simulink model "fromworkspace_test"  (Simulink 8.4)
settings: Solver=VariableStepDiscrete  StartTime=0.0  StopTime=5  MaxStep=1  RelTol=1e-3
settings Model: Creator=arnaud  LastModifiedBy=arnaud
settings DataIOCC: ExternalInput=xin  SaveFormat=Structure

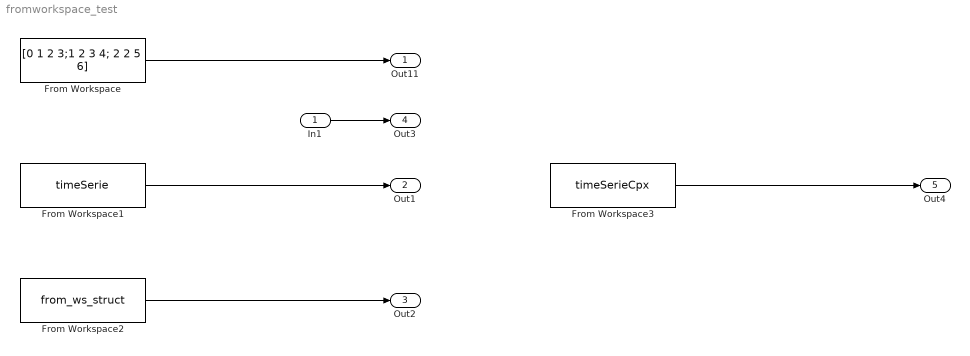
== system fromworkspace_test ==
  In1 : Inport
  From Workspace : FromWorkspace  VariableName=[0 1 2 3;1 2 3 4; 2 2 5 6]  SampleTime=0
  From Workspace1 : FromWorkspace  VariableName=timeSerie  SampleTime=0
  From Workspace2 : FromWorkspace  VariableName=from_ws_struct  OutDataTypeStr=double  SampleTime=0
  From Workspace3 : FromWorkspace  VariableName=timeSerieCpx  SampleTime=0
  Out11 : Outport
  Out1 : Outport  Port=2
  Out2 : Outport  Port=3
  Out3 : Outport  Port=4
  Out4 : Outport  Port=5
  wires:
  From Workspace/1 -> Out11/1
  From Workspace1/1 -> Out1/1
  From Workspace2/1 -> Out2/1
  In1/1 -> Out3/1
  From Workspace3/1 -> Out4/1
